simulink model "Isolated_ZVS_boost_converter"  (R2020a)
settings: Solver=VariableStepAuto  StartTime=0.0  StopTime=1  RelTol=1e-3  EnableMultiTasking=on
libraries: powerlib x15, simulink x1
settings Model: Creator=sunil  LastModifiedBy=sunil
settings DataIOCC: ReturnWorkspaceOutputs=off
settings OptimizationCC: LifeSpan=inf
settings DebuggingCC: SFUnexpectedBacktrackingDiag=warning  SFNoUnconditionalDefaultTransitionDiag=warning  ArithmeticOperatorsInVariantConditions=warning
settings SFSimCC: SimUseLocalCustomCode=off  CustomCodeUndefinedFunction=UseInterfaceOnly
settings RTWCC: RTWUseLocalCustomCode=off
settings CodeAppCC: StateflowObjectComments=on
settings GRTTargetCC: TargetLangStandard=C89/C90 (ANSI)
settings ConfigComp: CovMetricSettings=dw  CovHtmlReporting=on  CovSaveCumulativeToWorkspaceVar=on  CovSaveSingleToWorkspaceVar=on  CovExternalEMLEnable=off
settings SimscapeCC: SimscapeNormalizeSystem=off

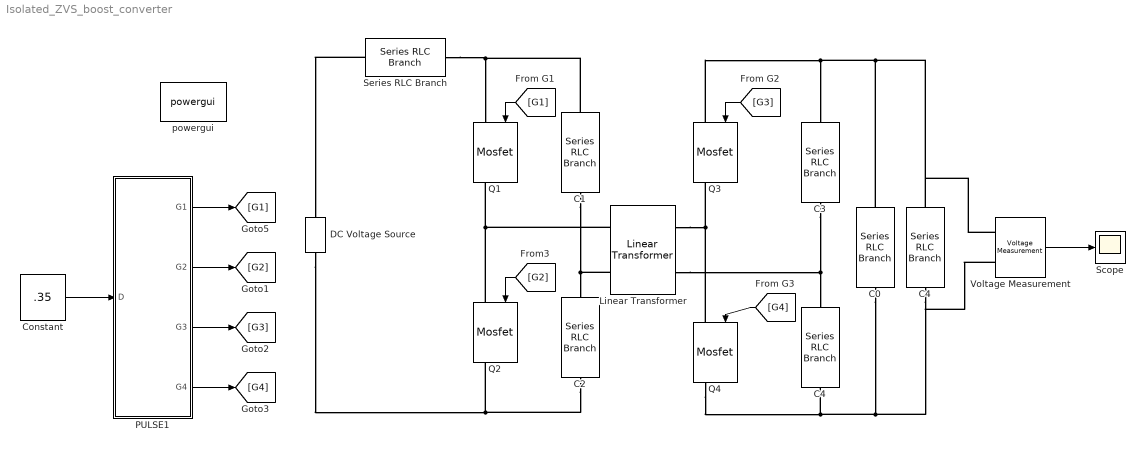
== system Isolated_ZVS_boost_converter ==
  "           C4" : powerlib/Elements/Series RLC Branch  LConnTagsString=__new0  RConnTagsString=__new0  BranchType=C  Resistance=1  Inductance=1e-3  SetiL0=off  InitialCurrent=0  Capacitance=10e-6  Setx0=off  InitialVoltage=0  Measurements=None
  C{0..3} (4 alike) : powerlib/Elements/Series RLC Branch  LConnTagsString=__new0  RConnTagsString=__new0  BranchType=C  Resistance=1  Inductance=1e-3  SetiL0=off  InitialCurrent=0  Capacitance=10e-6  Setx0=off  InitialVoltage=0  Measurements=None
  C4 : powerlib/Elements/Series RLC Branch  LConnTagsString=__new0  RConnTagsString=__new0  BranchType=R  Resistance=435  Inductance=1e-3  SetiL0=off  InitialCurrent=0  Capacitance=10e-6  Setx0=off  InitialVoltage=0  Measurements=None
  Constant : Constant  Value=.35
  DC Voltage Source : powerlib/Electrical Sources/DC Voltage Source  Amplitude=100  Measurements=None
  Linear Transformer : powerlib/Elements/Linear Transformer  UNITS=pu  NominalPower=[16000 50 ]  winding1="[100*1.414 .002  0.0005]"  winding2=[300*1.414 .002 0.0005]  ThreeWindings=off  winding3=[ 315e3 0.002 0.08 ]  RmLm=[ 500 500 ]  Measurements=None  DataType=off
  PULSE1 : Subsystem
  Q{1..4} (4 alike) : powerlib/Power Electronics/Mosfet  Ron=0.1  Lon=0  Rd=0.01  Vfd=0  IC=0  Rs=1e5  Cs=inf  Measurements=on
  Scope : Scope
  Series RLC Branch : powerlib/Elements/Series RLC Branch  LConnTagsString=__new0  RConnTagsString=__new0  BranchType=L  Resistance=1  Inductance=0.56e-6  SetiL0=off  InitialCurrent=0  Capacitance=1e-6  Setx0=off  InitialVoltage=0  Measurements=None
  Voltage Measurement : powerlib/Measurements/Voltage Measurement  PhasorSimulation=off  OutputType=Complex  PSBequivalent=0
  powergui : powerlib/powergui  Priority=1  SimulationMode=Discrete  SampleTime=5e-6  frequency=60  Iterations=50  frequencyindice=0  Pbase=100e6  ErrMax=1e-4  UnitsV=kV  UnitsW=MW  buscounter=0  FunctionMessages=off  echomessages=off  EnableUseOfTLC=off  CurrentSourceSwitches=off  DisableSnubberDevices=off  DisableRonSwitches=off  DisableVfSwitches=off  DisplayEquations=off  AutomaticDiscreteSolvers=off  SolverType=Tustin/Backward Euler (TBE)  Interpol=off  ExternalGateDelay=off  methode=off  Ts=10  x0status=blocks  SPID=off  SwTol=0  HookPort=off  NonlinearTolerance=1e-4  nMaxIteration=100  ContinueOnMaxIteration=off  RestoreLinks=warning  ResistiveCurrentMeasurement=off  Frange=[0:2:500]  Ylog=off  Xlog=on  ShowGrid=off  save=off  variable=ZData  structure=0  ZoomFFT=off  StartTime=0.0  cycles=1  DisplayStyle=1  fundamental=60  FreqAxis=off  MaxFrequency=1000  frequencyindicesteady=1  RmsSteady=1  display=off
  wires:
  PULSE1/2(G2) -> [G2]
  [G1] -> Q1/1
  [G4] -> Q4/1
  [G2] -> Q2/1
  [G3] -> Q3/1
  PULSE1/1(G1) -> [G1]
  Voltage Measurement/1 -> Scope/1
  Constant/1 -> PULSE1/1(D)
  PULSE1/3(G3) -> [G3]
  PULSE1/4(G4) -> [G4]
  connections:
  Series RLC Branch/RConn1 -- Q1/LConn1 -- C1/LConn1
  Series RLC Branch/LConn1 -- DC Voltage Source/RConn1
  DC Voltage Source/LConn1 -- C2/RConn1 -- Q2/RConn1
  C1/RConn1 -- Linear Transformer/LConn2 -- C2/LConn1
  Q2/LConn1 -- Linear Transformer/LConn1 -- Q1/RConn1
  Q4/LConn1 -- Q3/RConn1 -- Linear Transformer/RConn1
  Q3/LConn1 -- C4/LConn1 -- Voltage Measurement/LConn1 -- C0/LConn1 -- C3/LConn1
  C3/RConn1 -- Linear Transformer/RConn2 -- "           C4"/LConn1
  Q4/RConn1 -- C4/RConn1 -- Voltage Measurement/LConn2 -- C0/RConn1 -- "           C4"/RConn1

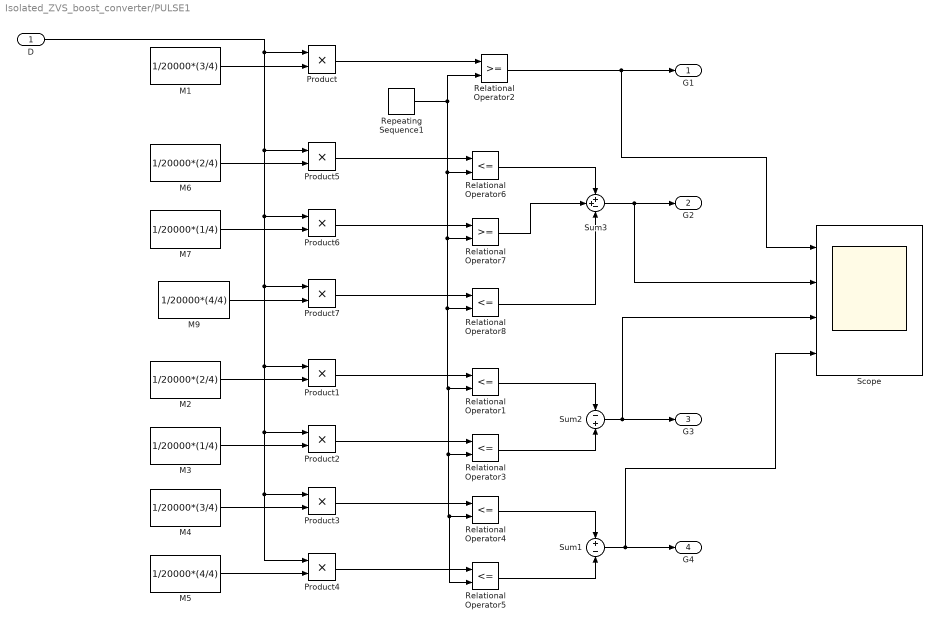
== system Isolated_ZVS_boost_converter/PULSE1 ==
  D : Inport
  M1 : Constant  Value=1/20000*(3/4)
  M2 : Constant  Value=1/20000*(2/4)
  M3 : Constant  Value=1/20000*(1/4)
  M4 : Constant  Value=1/20000*(3/4)
  M5 : Constant  Value=1/20000*(4/4)
  M6 : Constant  Value=1/20000*(2/4)
  M7 : Constant  Value=1/20000*(1/4)
  M9 : Constant  Value=1/20000*(4/4)
  Product{,1..7} (8 alike) : Product
  Relational Operator{1,3..6,8} (6 alike) : RelationalOperator  Operator=<=  OutDataTypeStr=boolean  RndMeth=Nearest
  Relational Operator2 : RelationalOperator  OutDataTypeStr=boolean  RndMeth=Nearest
  Relational Operator7 : RelationalOperator  OutDataTypeStr=boolean  RndMeth=Nearest
  Repeating Sequence1 : simulink/Sources/Repeating Sequence  rep_seq_t=[0 1/20000]  rep_seq_y=[0 1/20000]
  Scope : Scope  NumInputPorts=4
  Sum1 : Sum  Inputs=+-
  Sum2 : Sum  Inputs=-+
  Sum3 : Sum  Inputs=++-
  G1 : Outport
  G2 : Outport  Port=2
  G3 : Outport  Port=3
  G4 : Outport  Port=4
  wires:
  Relational Operator2/1 -> Scope/1, G1/1
  Sum3/1 -> Scope/2, G2/1
  Relational Operator6/1 -> Sum3/1
  M1/1 -> Product/2
  M7/1 -> Product6/2
  Product/1 -> Relational Operator2/1
  Product5/1 -> Relational Operator6/1
  M6/1 -> Product5/2
  Product6/1 -> Relational Operator7/1
  Repeating Sequence1/1 -> Relational Operator2/2, Relational Operator5/2, Relational Operator4/2, Relational Operator3/2, Relational Operator1/2, Relational Operator8/2, Relational Operator7/2, Relational Operator6/2
  M9/1 -> Product7/2
  Product7/1 -> Relational Operator8/1
  D/1 -> Product4/1, Product3/1, Product2/1, Product1/1, Product7/1, Product6/1, Product5/1, Product/1
  Relational Operator7/1 -> Sum3/2
  Relational Operator8/1 -> Sum3/3
  Sum2/1 -> Scope/3, G3/1
  Relational Operator1/1 -> Sum2/1
  Relational Operator4/1 -> Sum1/1
  Relational Operator5/1 -> Sum1/2
  Sum1/1 -> G4/1, Scope/4
  M2/1 -> Product1/2
  M3/1 -> Product2/2
  M4/1 -> Product3/2
  M5/1 -> Product4/2
  Product1/1 -> Relational Operator1/1
  Product2/1 -> Relational Operator3/1
  Product3/1 -> Relational Operator4/1
  Product4/1 -> Relational Operator5/1
  Relational Operator3/1 -> Sum2/2
